simulink model "plant_open_loop_step_steer_test"  (R2026a)
settings: Solver=VariableStepAuto
undefined symbols (not defined in the file): test_drive_torque_Nm, test_road_friction_mu, test_step_time_s
settings Model: Creator=rayyu  LastModifiedBy=rayyu

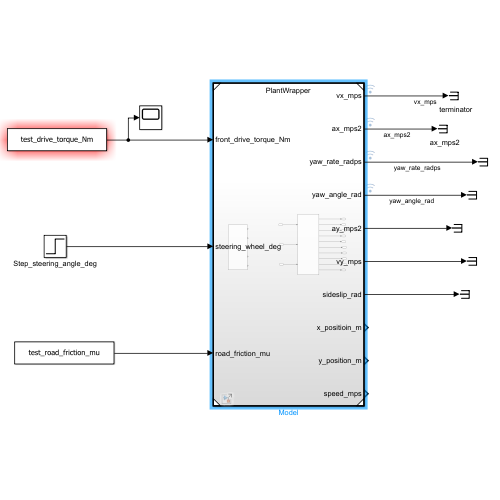
[thumbnail: Simulink's stored preview of the top-level diagram]
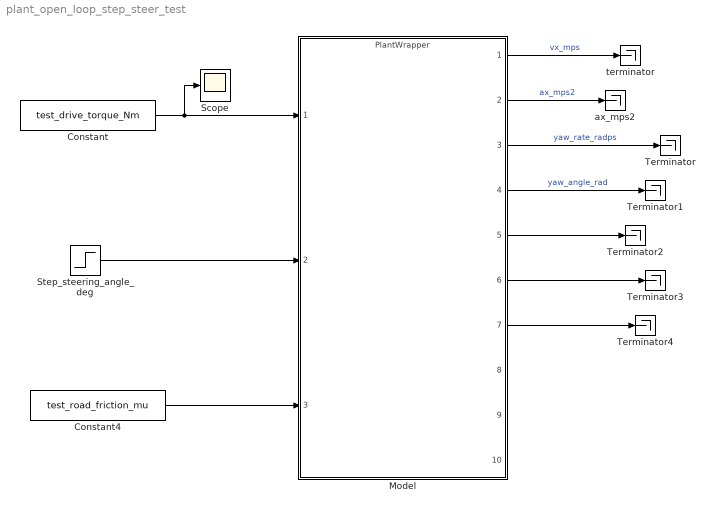
== system plant_open_loop_step_steer_test ==
  Constant : Constant  Value=test_drive_torque_Nm  VectorParams1D=off  SampleTime=0.01
  Constant4 : Constant  Value=test_road_friction_mu
  Model : ModelReference  ModelNameDialog=PlantWrapper.slx  SimulationMode=Normal  ModelReferenceVersion=1.16
  Scope : Scope
      settings: ActiveDisplayYMinimum=90  ActiveDisplayYMaximum=110
  Step_steering_angle_deg : Step  Time=test_step_time_s  FinalValue=test_steering_wheel_deg  SampleTime=0
  Terminator{,1..4} (5 alike) : Terminator
  ax_mps2 : Terminator
  terminator : Terminator
  wires:
  Model/2 -> ax_mps2/1  "ax_mps2"
  Model/7 -> Terminator4/1
  Constant/1 -> Scope/1, Model/1
  Model/5 -> Terminator2/1
  Model/3 -> Terminator/1  "yaw_rate_radps"
  Model/6 -> Terminator3/1
  Model/4 -> Terminator1/1  "yaw_angle_rad"
  Constant4/1 -> Model/3
  Model/1 -> terminator/1  "vx_mps"
  Step_steering_angle_deg/1 -> Model/2
